simulink model "two_link_extended_force"  (R2022b)
settings: Solver=VariableStepAuto  StartTime=0.0  StopTime=10.0  RelTol=1e-3
values from neighbouring files (symbols this model uses):
  a_1 = 1    [parameters.m]
  a_2 = 1    [parameters.m]
  F = [0.1, 0 ... (first row only)    [parameters.m]
  init = [0.75*pi;-0.75*pi]    [parameters.m]
  kx = 100    [parameters.m]
  xr = 0.5    [parameters.m]
settings Model: Creator=eleves  LastModifiedBy=eleves
settings ModelReferenceCC: ModelReferenceMinAlgLoopOccurrences=on

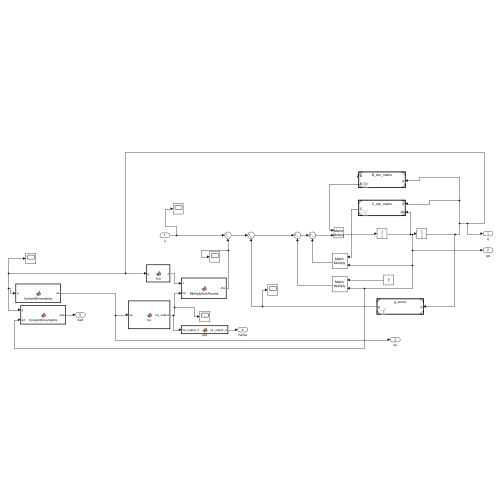
[thumbnail: Simulink's stored preview of the top-level diagram]
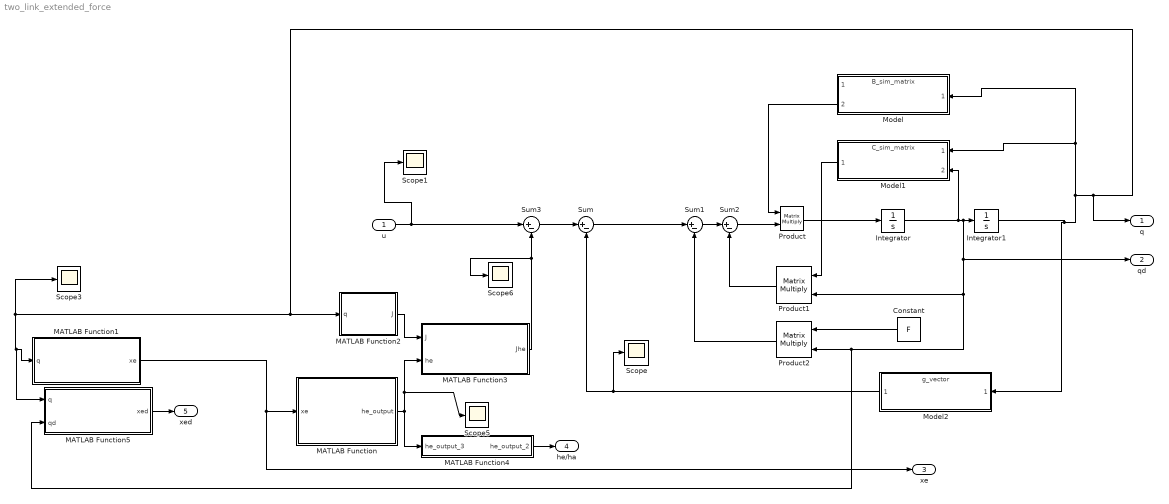
== system two_link_extended_force ==
  u : Inport  PortDimensions=2
  Constant : Constant  Value=F
  Integrator : Integrator
  Integrator1 : Integrator  InitialCondition=init
  MATLAB Function : MATLAB Function  TreatAsAtomicUnit=on
  MATLAB Function1 : MATLAB Function  TreatAsAtomicUnit=on
  MATLAB Function2 : MATLAB Function  TreatAsAtomicUnit=on
  MATLAB Function3 : MATLAB Function  TreatAsAtomicUnit=on
  MATLAB Function4 : MATLAB Function  TreatAsAtomicUnit=on
  MATLAB Function5 : MATLAB Function  TreatAsAtomicUnit=on
  Model : ModelReference  ModelNameDialog=B_sim_matrix.slx  SimulationMode=Normal  ModelReferenceVersion=13.0
  Model1 : ModelReference  ModelNameDialog=C_sim_matrix.slx  SimulationMode=Normal  ModelReferenceVersion=1.2
  Model2 : ModelReference  ModelNameDialog=g_vector.slx  SimulationMode=Normal  ModelReferenceVersion=1.8
  Product : Product  Multiplication=Matrix(*)
  Product1 : Product  Multiplication=Matrix(*)
  Product2 : Product  Multiplication=Matrix(*)
  Scope{,1,3,5..6} (5 alike) : Scope
  Sum{,1..3} (4 alike) : Sum  Inputs=|+-
  q : Outport  PortDimensions=2
  qd : Outport  Port=2  PortDimensions=2
  xe : Outport  Port=3  PortDimensions=2
  he/ha : Outport  Port=4  PortDimensions=2
  xed : Outport  Port=5  PortDimensions=2
  wires:
  MATLAB Function4/1(he_output_2) -> he/ha/1
  Product/1 -> Integrator/1
  Sum1/1 -> Sum2/1
  Integrator1/1 -> Model2/1, Model/1, Model1/1, MATLAB Function5/1(q), MATLAB Function1/1(q), Scope3/1, MATLAB Function2/1(q), q/1
  u/1 -> Sum3/1, Scope1/1
  Sum3/1 -> Sum/1
  MATLAB Function2/1(J) -> MATLAB Function3/1(J)
  Product2/1 -> Sum1/2
  Product1/1 -> Sum2/2
  Sum/1 -> Sum1/1
  MATLAB Function/1(he_output) -> MATLAB Function4/1(he_output_3), MATLAB Function3/2(he), Scope5/1
  Model/2 -> Product/1
  Model2/1 -> Scope/1, Sum/2
  Constant/1 -> Product2/1
  Sum2/1 -> Product/2
  MATLAB Function1/1(xe) -> xe/1, MATLAB Function/1(xe)
  MATLAB Function3/1(Jhe) -> Scope6/1, Sum3/2
  Model1/1 -> Product1/1
  Integrator/1 -> Model1/2, qd/1, MATLAB Function5/2(qd), Product2/2, Product1/2, Integrator1/1
  MATLAB Function5/1(xed) -> xed/1

== matlab function two_link_extended_force/MATLAB Function1 ==
  data: q input; xe output; a_1 parameter; a_2 parameter
function xe  = forwardKinematics(q,a_1, a_2)

    t1 = q(1);
    t2 = q(2);
    t12 = t1+t2;
    ct1 = cos(t1);
    ct12 = cos(t1+t2);
    st1 = sin(t1);
    st12 = sin(t2+t1);
    
%     To3 = [ cos(t1+t2),-sin(t1+t2),0,a_1*cos(t1)+a_2*cos(t1+t2);
%             sin(t1+t2),cos(t1+t2),0,a_1*sin(t1)+a_2*sin(t1+t2);
%             0,0,1,0;
%             0,0,0,1];
% %     T3e = [0,0,1,0;
% %             0,1,0,0;
% %             -1,0,0,0;
% %             0,0,0,1];
% %     
% %     T = To3*T3e;

    xe = [a_1*ct1+a_2*ct12;
        a_1*st1+a_2*st12];

   
    
end

== matlab function two_link_extended_force/MATLAB Function ==
  data: xe input; he_output output; xr parameter; kx parameter
function he_output  = he(xe,xr,kx)
    he_output_scalar = 0;    
    xe = xe(1);
    if xe >= xr
        he_output_scalar = kx*(xe-xr);
    end

    he_output_line = [he_output_scalar,0,0];
    he_output = transpose(he_output_line);
end

== matlab function two_link_extended_force/MATLAB Function2 ==
  data: q input; J output; a_1 parameter; a_2 parameter
function J = fcn(q, a_1, a_2)
    theta1 = q(1);
    theta2 = q(2);
    J = [-a_1*sin(theta1)-a_2*sin(theta1+theta2),-a_2*sin(theta1+theta2),0;
        a_1*cos(theta1)+a_2*cos(theta1+theta2),a_2*cos(theta1+theta2),0;
        0,0,0;
        0,0,0;
        0,0,0;
        1,1,1;];

end

== matlab function two_link_extended_force/MATLAB Function3 ==
  data: J input; Jhe output; he input
function Jhe = MultiplyAndAccess(J,he)
    J = transpose(J(1:2,1:2));
    he = he(1:2,1);
    Jhetemp = J*he;
    Jhe = Jhetemp(1:2,1);
end

== matlab function two_link_extended_force/MATLAB Function4 ==
  data: he_output_3 input; he_output_2 output
function he_output_2  = red(he_output_3)
    he_output_2 = [he_output_3(1);he_output_3(2)];
end

== matlab function two_link_extended_force/MATLAB Function5 ==
  data: q input; qd input; xed output; a_1 parameter; a_2 parameter
function xed  = forwardKinematics(q,qd,a_1, a_2)

    t1 = q(1);
    t2 = q(2);
    t12 = t1+t2;
    t1d = qd(1);
    t12d = qd(1)+qd(2);
    ct1 = cos(t1);
    ct12 = cos(t1+t2);
    st1 = sin(t1);
    st12 = sin(t2+t1);
    
%     To3 = [ cos(t1+t2),-sin(t1+t2),0,a_1*cos(t1)+a_2*cos(t1+t2);
%             sin(t1+t2),cos(t1+t2),0,a_1*sin(t1)+a_2*sin(t1+t2);
%             0,0,1,0;
%             0,0,0,1];
% %     T3e = [0,0,1,0;
% %             0,1,0,0;
% %             -1,0,0,0;
% %             0,0,0,1];
% %     
% %     T = To3*T3e;

    xed = [-a_1*t1d*st1-a_2*t12d*st12;
        a_1*t1d*ct1+a_2*t12d*ct12];

   
    
end
